simulink model "Mode_plus_Longitudinal"  (R2015a)
settings: Solver=ode45  StartTime=0.0  StopTime=10.0  RelTol=1e-3
undefined symbols (not defined in the file): dt, sample
libraries: simulink x10
settings Model: CovSFcnEnable=off  Creator=teme  LastModifiedBy=teme
settings DataIOCC: SaveFormat=Structure
settings DebuggingCC: UnderspecifiedInitializationDetection=Classic  MergeDetectMultiDrivingBlocksExec=none  SolverPrmCheckMsg=warning  StateNameClashWarn=warning

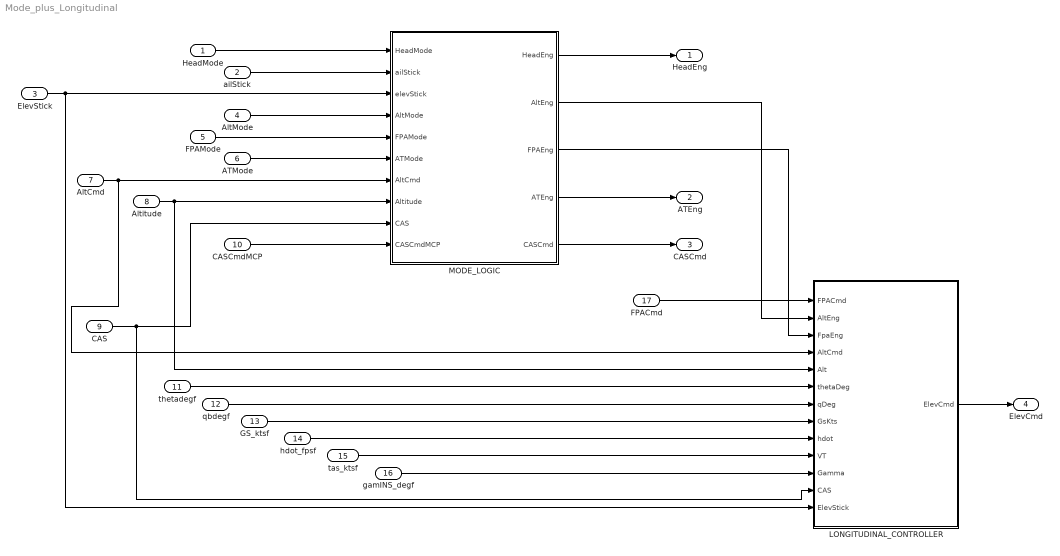
== system Mode_plus_Longitudinal ==
  HeadMode : Inport
  ailStick : Inport  Port=2
  ElevStick : Inport  Port=3
  AltMode : Inport  Port=4
  FPAMode : Inport  Port=5
  ATMode : Inport  Port=6
  AltCmd : Inport  Port=7
  Altitude : Inport  Port=8
  CAS : Inport  Port=9
  CASCmdMCP : Inport  Port=10
  thetadegf : Inport  Port=11  OutDataTypeStr=double
  qbdegf : Inport  Port=12  OutDataTypeStr=double
  GS_ktsf : Inport  Port=13  OutDataTypeStr=double
  "hdot_fpsf " : Inport  Port=14  OutDataTypeStr=double
  tas_ktsf : Inport  Port=15  OutDataTypeStr=double
  gamINS_degf : Inport  Port=16  OutDataTypeStr=double
  FPACmd : Inport  Port=17  OutDataTypeStr=double
  LONGITUDINAL_CONTROLLER : Subsystem  TreatAsAtomicUnit=on
  MODE_LOGIC : Subsystem  TreatAsAtomicUnit=on
  HeadEng : Outport
  ATEng : Outport  Port=2
  CASCmd : Outport  Port=3
  ElevCmd : Outport  RequirementInfo={} %GIDa_1472b341_5948_49bd_8afc_f716c029507f  Port=4
  wires:
  HeadMode/1 -> MODE_LOGIC/1(HeadMode)
  ailStick/1 -> MODE_LOGIC/2(ailStick)
  AltMode/1 -> MODE_LOGIC/4(AltMode)
  FPAMode/1 -> MODE_LOGIC/5(FPAMode)
  ATMode/1 -> MODE_LOGIC/6(ATMode)
  CASCmdMCP/1 -> MODE_LOGIC/10(CASCmdMCP)
  MODE_LOGIC/1(HeadEng) -> HeadEng/1
  MODE_LOGIC/2(AltEng) -> LONGITUDINAL_CONTROLLER/2(AltEng)
  MODE_LOGIC/3(FPAEng) -> LONGITUDINAL_CONTROLLER/3(FpaEng)
  MODE_LOGIC/4(ATEng) -> ATEng/1
  MODE_LOGIC/5(CASCmd) -> CASCmd/1
  LONGITUDINAL_CONTROLLER/1(ElevCmd) -> ElevCmd/1
  CAS/1 -> MODE_LOGIC/9(CAS), LONGITUDINAL_CONTROLLER/12(CAS)
  FPACmd/1 -> LONGITUDINAL_CONTROLLER/1(FPACmd)
  AltCmd/1 -> LONGITUDINAL_CONTROLLER/4(AltCmd), MODE_LOGIC/7(AltCmd)
  Altitude/1 -> MODE_LOGIC/8(Altitude), LONGITUDINAL_CONTROLLER/5(Alt)
  thetadegf/1 -> LONGITUDINAL_CONTROLLER/6(thetaDeg)
  qbdegf/1 -> LONGITUDINAL_CONTROLLER/7(qDeg)
  GS_ktsf/1 -> LONGITUDINAL_CONTROLLER/8(GsKts)
  "hdot_fpsf "/1 -> LONGITUDINAL_CONTROLLER/9(hdot)
  tas_ktsf/1 -> LONGITUDINAL_CONTROLLER/10(VT)
  gamINS_degf/1 -> LONGITUDINAL_CONTROLLER/11(Gamma)
  ElevStick/1 -> LONGITUDINAL_CONTROLLER/13(ElevStick), MODE_LOGIC/3(elevStick)

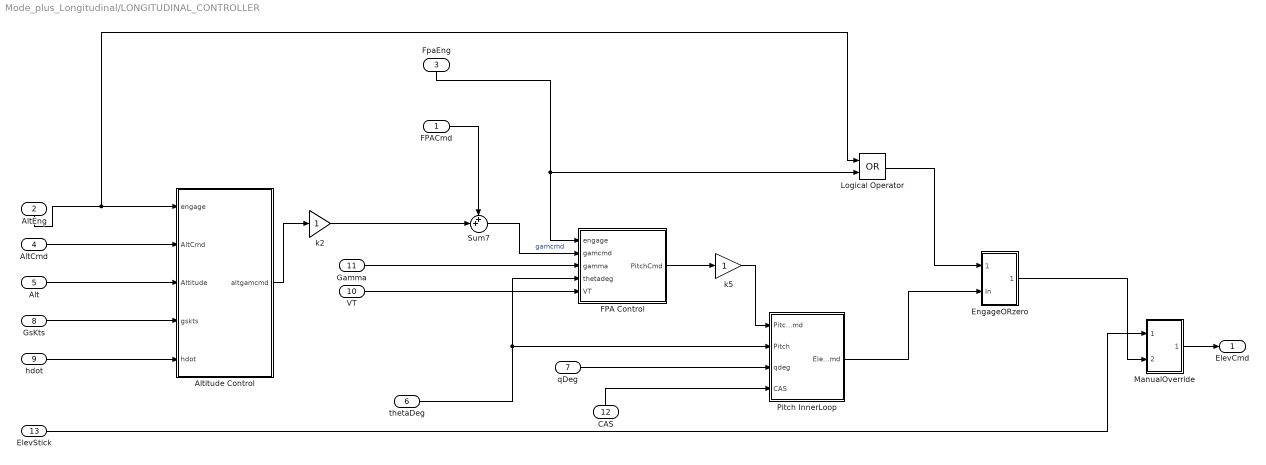
== system Mode_plus_Longitudinal/LONGITUDINAL_CONTROLLER ==
  FPACmd : Inport
  AltEng : Inport  Port=2
  FpaEng : Inport  Port=3
  AltCmd : Inport  Port=4
  Alt : Inport  Port=5
  thetaDeg : Inport  Port=6
  qDeg : Inport  Port=7
  GsKts : Inport  Port=8
  hdot : Inport  Port=9
  VT : Inport  Port=10
  Gamma : Inport  Port=11
  CAS : Inport  Port=12
  ElevStick : Inport  Port=13
  Altitude Control : Subsystem  RequirementInfo={'other' '..\..\tcm_requirements.docx' '@Simulink_requirement_item_14' 'true' 'Altitude Control' '' } %GIDa_355d9ec8_0b7f_4143_baa6_003c4a27f8c0  TreatAsAtomicUnit=on
  EngageORzero : Subsystem  TreatAsAtomicUnit=on
  FPA Control : Subsystem  RequirementInfo={'other' '..\..\tcm_requirements.docx' '@Simulink_requirement_item_15' 'true' 'FPA Control' '' } %GIDa_afe01289_fe8a_4a07_8f72_45e0944c7946  TreatAsAtomicUnit=on
  Logical Operator : Logic  Operator=OR  AllPortsSameDT=off  OutDataTypeStr=boolean
  ManualOverride : Subsystem  TreatAsAtomicUnit=on
  Pitch InnerLoop : Subsystem  RequirementInfo={'other' '..\..\tcm_requirements.docx' '@Simulink_requirement_item_17' 'true' 'Pitch InnerLoop' '' } %GIDa_d1872e6f_e306_4912_a3b7_97524d87ca2c  TreatAsAtomicUnit=on
  Sum7 : Sum  RequirementInfo={} %GIDa_0c140ded_69fd_4573_8acf_9eb9bb189775  Inputs=++|
  k2 : Gain  RequirementInfo={} %GIDa_583ddfee_05b2_4a69_b1d4_b6583806e97d
  k5 : Gain  RequirementInfo={} %GIDa_c5e5a863_50d1_4c0f_a080_0e1eca729c49
  ElevCmd : Outport
  wires:
  k2/1 -> Sum7/2
  Alt/1 -> Altitude Control/3(Altitude)
  thetaDeg/1 -> Pitch InnerLoop/2(Pitch), FPA Control/4(thetadeg)
  Gamma/1 -> FPA Control/3(gamma)
  AltCmd/1 -> Altitude Control/2(AltCmd)
  ManualOverride/1(Out) -> ElevCmd/1
  Altitude Control/1(altgamcmd) -> k2/1
  FPA Control/1(PitchCmd) -> k5/1
  hdot/1 -> Altitude Control/5(hdot)
  Sum7/1 -> FPA Control/2(gamcmd)  "gamcmd"
  qDeg/1 -> Pitch InnerLoop/3(qdeg)
  GsKts/1 -> Altitude Control/4(gskts)
  VT/1 -> FPA Control/5(VT)
  FPACmd/1 -> Sum7/1
  k5/1 -> Pitch InnerLoop/1(PitchCmd)
  FpaEng/1 -> FPA Control/1(engage), Logical Operator/2
  CAS/1 -> Pitch InnerLoop/4(CAS)
  AltEng/1 -> Logical Operator/1, Altitude Control/1(engage)
  ElevStick/1 -> ManualOverride/1(Man)
  Pitch InnerLoop/1(ElevCmd) -> EngageORzero/2(In)
  EngageORzero/1(Out) -> ManualOverride/2(Auto)
  Logical Operator/1 -> EngageORzero/1(Engage)

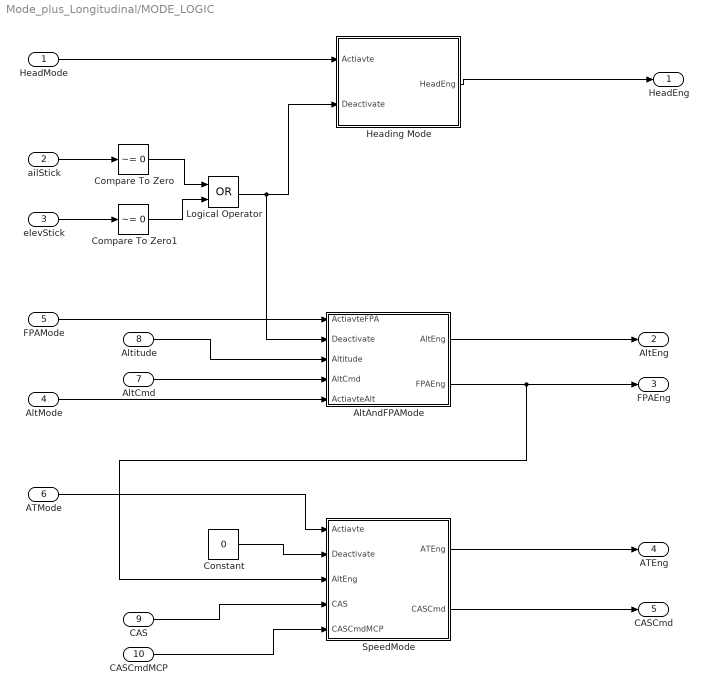
== system Mode_plus_Longitudinal/MODE_LOGIC ==
  HeadMode : Inport
  ailStick : Inport  Port=2
  elevStick : Inport  Port=3
  AltMode : Inport  Port=4
  FPAMode : Inport  Port=5
  ATMode : Inport  Port=6
  AltCmd : Inport  Port=7
  Altitude : Inport  Port=8
  CAS : Inport  Port=9
  CASCmdMCP : Inport  Port=10
  AltAndFPAMode : Subsystem  TreatAsAtomicUnit=on
  Compare To Zero : simulink/Logic and Bit Operations/Compare To Zero  relop=~=  OutDataTypeStr=boolean
  Compare To Zero1 : simulink/Logic and Bit Operations/Compare To Zero  relop=~=  OutDataTypeStr=boolean
  Constant : Constant  Value=0
  Heading Mode : Subsystem  TreatAsAtomicUnit=on
  Logical Operator : Logic  Operator=OR  AllPortsSameDT=off  OutDataTypeStr=boolean
  SpeedMode : Subsystem  TreatAsAtomicUnit=on
  HeadEng : Outport
  AltEng : Outport  Port=2
  FPAEng : Outport  Port=3
  ATEng : Outport  Port=4
  CASCmd : Outport  Port=5
  wires:
  SpeedMode/1(ATEng) -> ATEng/1
  ailStick/1 -> Compare To Zero/1
  Constant/1 -> SpeedMode/2(Deactivate)
  AltAndFPAMode/2(FPAEng) -> FPAEng/1, SpeedMode/3(AltEng)
  AltAndFPAMode/1(AltEng) -> AltEng/1
  Heading Mode/1(HeadEng) -> HeadEng/1
  HeadMode/1 -> Heading Mode/1(Actiavte)
  Compare To Zero1/1 -> Logical Operator/2
  Compare To Zero/1 -> Logical Operator/1
  elevStick/1 -> Compare To Zero1/1
  ATMode/1 -> SpeedMode/1(Actiavte)
  FPAMode/1 -> AltAndFPAMode/1(ActiavteFPA)
  Altitude/1 -> AltAndFPAMode/3(Altitude)
  AltMode/1 -> AltAndFPAMode/5(ActiavteAlt)
  Logical Operator/1 -> AltAndFPAMode/2(Deactivate), Heading Mode/2(Deactivate)
  CASCmdMCP/1 -> SpeedMode/5(CASCmdMCP)
  AltCmd/1 -> AltAndFPAMode/4(AltCmd)
  SpeedMode/2(CASCmd) -> CASCmd/1
  CAS/1 -> SpeedMode/4(CAS)

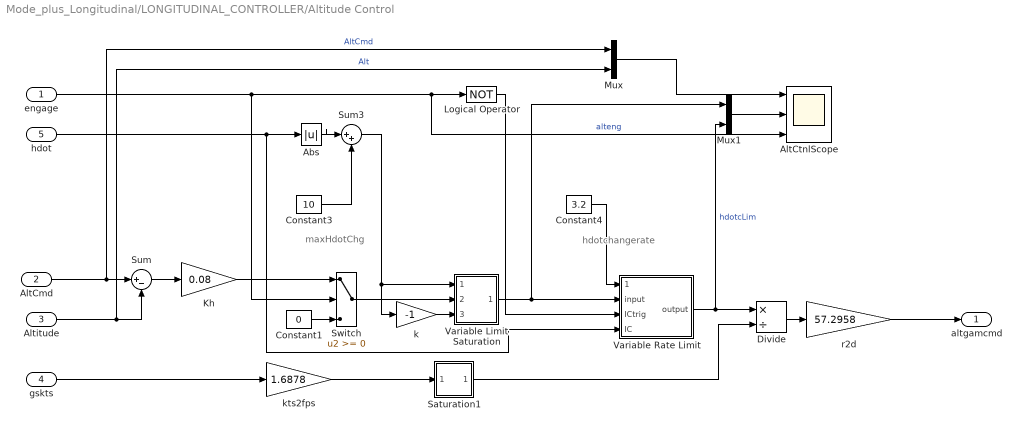
== system Mode_plus_Longitudinal/LONGITUDINAL_CONTROLLER/Altitude Control ==
  note: hdotchangerate
  note: maxHdotChg
  engage : Inport  RequirementInfo={} %GIDa_52c363b5_d7dd_4428_9d3d_bb77c4e76d98
  AltCmd : Inport  RequirementInfo={} %GIDa_0a82d765_f654_4276_830a_f6372a89bbe0  Port=2
  Altitude : Inport  RequirementInfo={} %GIDa_e8d70308_bc0e_4fcb_b765_d7e59f7ec592  Port=3
  gskts : Inport  RequirementInfo={} %GIDa_2af44391_9073_42ae_9a32_99820c2e56f5  Port=4
  hdot : Inport  RequirementInfo={} %GIDa_d9b9fdf0_6dc0_451b_abea_72e0c7ba7654  Port=5
  Abs : Abs  RequirementInfo={} %GIDa_dbe4ef0d_0270_47f9_8208_b0358621302e  SaturateOnIntegerOverflow=on
  AltCtnlScope : Scope  NumInputPorts=3
      settings: RequirementInfo={} %GIDa_cdbaa36f_c6c9_4411_8b52_1b5689d7b849  TimeRange=30  YMin=10000~-5~0  YMax=10200~15~1  SaveName=ScopeData3
  Constant1 : Constant  RequirementInfo={} %GIDa_a96aea24_dc3f_4446_af9b_51dc29300d52  Value=0
  Constant3 : Constant  RequirementInfo={} %GIDa_b1d1ceb1_281f_4f1b_8837_6dd68452e06f  Value=10
  Constant4 : Constant  RequirementInfo={} %GIDa_a7351357_5fac_4e27_bfae_0a136a455002  Value=3.2
  Divide : Product  RequirementInfo={} %GIDa_b8ce34ec_9450_4665_b60e_f19377b61b94  Inputs=*/
  Kh : Gain  RequirementInfo={} %GIDa_2cbc3e69_edde_4cac_a935_06834fe77e88  Gain=0.08
  Logical Operator : Logic  RequirementInfo={} %GIDa_af0e9a41_cde9_4810_9311_1f14359ef5fb  Operator=NOT
  Mux : Mux  RequirementInfo={} %GIDa_47470e8e_2f36_4b9c_b2c4_1f6b7143c7a9  Inputs=2
  Mux1 : Mux  RequirementInfo={} %GIDa_61bb53ed_7736_48c8_9e72_c55612e66728  Inputs=2
  Saturation1 : Subsystem  RequirementInfo={} %GIDa_e76216f3_4aa2_40a0_8972_6dea82147eb2  TreatAsAtomicUnit=on
  Sum : Sum  RequirementInfo={} %GIDa_fdfab13b_0798_40e8_9730_db934c25849e  Inputs=|+-
  Sum3 : Sum  RequirementInfo={} %GIDa_64961105_2569_4900_8a9c_cb8f762adaeb  Inputs=|++  SaturateOnIntegerOverflow=on  InputSameDT=on  OutDataTypeStr=Inherit: Same as first input
  Switch : Switch  RequirementInfo={} %GIDa_2f10cc13_12cd_4e9c_841c_6addbf2a5c41
  Variable Rate Limit : Subsystem  RequirementInfo={} %GIDa_28bb6084_340d_4503_85e9_38193e023d28  TreatAsAtomicUnit=on
  Variable Limit Saturation : Subsystem  RequirementInfo={} %GIDa_69ead1b7_c762_43d5_aef2_f2ccefa8a597  TreatAsAtomicUnit=on
  k : Gain  RequirementInfo={} %GIDa_093f7639_44de_47ca_a1a9_8335a2ae5ad0  Gain=-1
  kts2fps : Gain  RequirementInfo={} %GIDa_c8935b0a_448f_434e_a3c9_42f3e55e9d5b  Gain=1.6878
  r2d : Gain  RequirementInfo={} %GIDa_7be9f1d5_d29b_4985_9ae9_ad523edcc485  Gain=57.2958
  altgamcmd : Outport  RequirementInfo={} %GIDa_a9afaf6f_4f56_4b87_9d4f_e24f69e92c68
  wires:
  Sum/1 -> Kh/1
  AltCmd/1 -> Sum/1, Mux/1  "AltCmd"
  Altitude/1 -> Sum/2, Mux/2  "Alt"
  hdot/1 -> Variable Rate Limit/4(IC), Abs/1
  Abs/1 -> Sum3/1
  Constant3/1 -> Sum3/2
  k/1 -> Variable Limit Saturation/3(Lo_lim)
  Sum3/1 -> k/1, Variable Limit Saturation/1(up_lim)
  engage/1 -> Switch/2, Logical Operator/1, AltCtnlScope/3  "alteng"
  gskts/1 -> kts2fps/1
  Divide/1 -> r2d/1
  r2d/1 -> altgamcmd/1
  Logical Operator/1 -> Variable Rate Limit/3(ICtrig)
  Variable Limit Saturation/1(Out1) -> Variable Rate Limit/2(input), Mux1/1
  Constant4/1 -> Variable Rate Limit/1(ratelim)
  Variable Rate Limit/1(output) -> Divide/1, Mux1/2  "hdotcLim"
  kts2fps/1 -> Saturation1/1(SigIn)
  Saturation1/1(Out1) -> Divide/2
  Switch/1 -> Variable Limit Saturation/2(SigIn)
  Kh/1 -> Switch/1
  Constant1/1 -> Switch/3
  Mux/1 -> AltCtnlScope/1
  Mux1/1 -> AltCtnlScope/2

== system Mode_plus_Longitudinal/LONGITUDINAL_CONTROLLER/EngageORzero ==
  Engage : Inport
  In : Inport  Port=2
  Logical Operator5 : Logic  RequirementInfo={} %GIDa_ccfc23e2_0411_4b04_aca7_2de4f158b6cd  AllPortsSameDT=off  OutDataTypeStr=boolean
  Switch1 : Switch  RequirementInfo={} %GIDa_254e92ee_ae0a_4bfe_bfdb_e4c06df78b5d  Threshold=0.5
  zero10 : Constant  RequirementInfo={} %GIDa_d207173f_5f9f_4849_a51b_8675c5c4c9c2
  zero9 : Constant  RequirementInfo={} %GIDa_ffbd3266_7e8f_4b22_959a_f4ffeace0558  Value=0
  Out : Outport
  wires:
  Engage/1 -> Logical Operator5/1
  zero10/1 -> Logical Operator5/2
  zero9/1 -> Switch1/3
  In/1 -> Switch1/1
  Logical Operator5/1 -> Switch1/2
  Switch1/1 -> Out/1

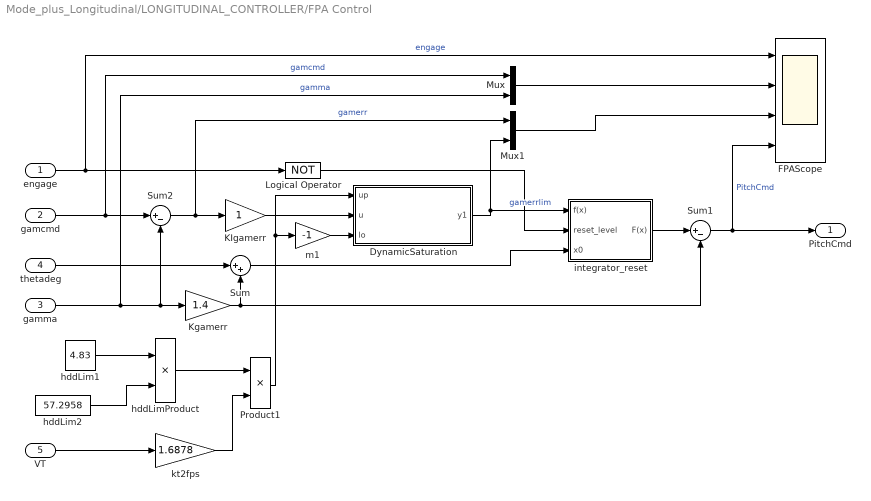
== system Mode_plus_Longitudinal/LONGITUDINAL_CONTROLLER/FPA Control ==
  engage : Inport  RequirementInfo={} %GIDa_a5ca5c72_1624_4f57_8848_6838dbeb69e5  OutDataTypeStr=boolean
  gamcmd : Inport  RequirementInfo={} %GIDa_f539d9e5_1422_4ddf_9938_0897544f30cd  Port=2  OutDataTypeStr=double
  gamma : Inport  RequirementInfo={} %GIDa_e241222a_57fb_4f96_ba9f_1fd449c16db7  Port=3  OutDataTypeStr=double
  thetadeg : Inport  RequirementInfo={} %GIDa_3c46ec82_f68a_45df_8609_de83facd241a  Port=4  OutDataTypeStr=double
  VT : Inport  RequirementInfo={} %GIDa_d515a720_002f_4829_a2a6_18045b0ac777  Port=5  OutDataTypeStr=double
  DynamicSaturation : Subsystem  TreatAsAtomicUnit=on
  FPAScope : Scope  NumInputPorts=4
      settings: RequirementInfo={} %GIDa_7cc530c8_9ccc_4bfe_b80a_f4375f56bd14  YMin=-1~-5~-2~-5  YMax=2~5~2~10
  KIgamerr : Gain  RequirementInfo={} %GIDa_82260f55_a1de_42fb_b735_9e4599f81841
  Kgamerr : Gain  RequirementInfo={} %GIDa_16083332_5456_45f2_a369_a033765805fc  Gain=1.4
  Logical Operator : Logic  RequirementInfo={} %GIDa_f4beb439_5138_4af2_9bd0_3d7cb852e6ec  Operator=NOT  AllPortsSameDT=off  OutDataTypeStr=boolean
  Mux : Mux  RequirementInfo={} %GIDa_f4a4be95_68e7_4fcc_80ef_d6f12325c5c6  Inputs=2
  Mux1 : Mux  RequirementInfo={} %GIDa_856a70e5_571d_4800_b63e_8744bb9a992b  Inputs=2
  Product1 : Product  RequirementInfo={} %GIDa_8e2f5a82_1404_4ef2_8700_b1676a09c733  RndMeth=Zero
  Sum : Sum  RequirementInfo={} %GIDa_2c46e54a_16c3_48c1_a530_4e77b3b6f7cf  Inputs=|++
  Sum1 : Sum  RequirementInfo={} %GIDa_5447bb63_ee33_484d_a3fb_66639f30e65e  Inputs=|+-
  Sum2 : Sum  RequirementInfo={} %GIDa_e6a645c9_6b06_4015_88ce_f90087de6b14  Inputs=|+-
  hddLim1 : Constant  Value=4.83  SampleTime=sample
  hddLim2 : Constant  Value=57.2958  SampleTime=sample
  hddLimProduct : Product  RndMeth=Zero
  integrator_reset : Subsystem  TreatAsAtomicUnit=on
  kt2fps : Gain  RequirementInfo={} %GIDa_e958a29f_6566_4fb6_a607_06b409395c8a  Gain=1.6878
  m1 : Gain  RequirementInfo={} %GIDa_f600f599_b9eb_4aa5_a121_c23ac8246818  Gain=-1
  PitchCmd : Outport  RequirementInfo={} %GIDa_7642116b_0bfd_4af5_a213_a8cf8bf5662a  OutDataTypeStr=double
  wires:
  Sum1/1 -> PitchCmd/1, FPAScope/4  "PitchCmd"
  Kgamerr/1 -> Sum1/2, Sum/2
  integrator_reset/1(F(x)) -> Sum1/1
  gamma/1 -> Kgamerr/1, Sum2/2, Mux/2  "gamma"
  thetadeg/1 -> Sum/1
  Sum/1 -> integrator_reset/3(x0)
  engage/1 -> Logical Operator/1, FPAScope/1  "engage"
  Logical Operator/1 -> integrator_reset/2(reset_level)
  kt2fps/1 -> Product1/2
  hddLimProduct/1 -> Product1/1
  Product1/1 -> m1/1, DynamicSaturation/1(up)
  VT/1 -> kt2fps/1
  DynamicSaturation/1(y1) -> integrator_reset/1(f(x)), Mux1/2  "gamerrlim"
  KIgamerr/1 -> DynamicSaturation/2(u)
  m1/1 -> DynamicSaturation/3(lo)
  Sum2/1 -> KIgamerr/1, Mux1/1  "gamerr"
  gamcmd/1 -> Sum2/1, Mux/1  "gamcmd"
  Mux/1 -> FPAScope/2
  Mux1/1 -> FPAScope/3
  hddLim1/1 -> hddLimProduct/1
  hddLim2/1 -> hddLimProduct/2

== system Mode_plus_Longitudinal/LONGITUDINAL_CONTROLLER/ManualOverride ==
  Man : Inport
  Auto : Inport  Port=2
  Switch1 : Switch  RequirementInfo={} %GIDa_69cd44cc_695c_4e4c_b729_5e76b03a5c9b  Criteria=u2 ~= 0  Threshold=0.5
  Out : Outport
  wires:
  Man/1 -> Switch1/3, Switch1/2
  Auto/1 -> Switch1/1
  Switch1/1 -> Out/1

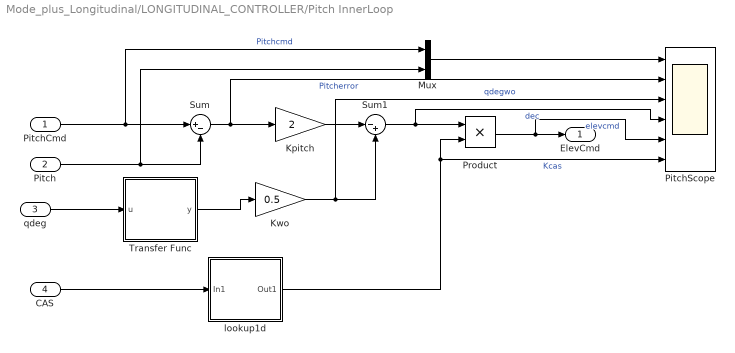
== system Mode_plus_Longitudinal/LONGITUDINAL_CONTROLLER/Pitch InnerLoop ==
  PitchCmd : Inport  RequirementInfo={} %GIDa_2fa8ae42_3276_495e_b4da_5cc7558fe53e  OutDataTypeStr=double
  Pitch : Inport  RequirementInfo={} %GIDa_e0b05770_7d89_48ca_ae42_7e8bc3cf70e1  Port=2  OutDataTypeStr=double
  qdeg : Inport  RequirementInfo={} %GIDa_32a3f04f_fa35_48b7_ae05_62ba74ce8106  Port=3  OutDataTypeStr=double
  CAS : Inport  RequirementInfo={} %GIDa_376f2873_f9f7_4b29_ab34_f3040502ee08  Port=4  OutDataTypeStr=double
  Kpitch : Gain  RequirementInfo={} %GIDa_7fbbd552_ea5b_4045_aa48_b875de2b9e68  Gain=2
  Kwo : Gain  RequirementInfo={} %GIDa_e54031bb_ac6b_45ac_907a_c4f2d5dd216d  Gain=0.5
  Mux : Mux  RequirementInfo={} %GIDa_2fd7bb9e_bac2_4662_8409_53cd9298505a  Inputs=2
  PitchScope : Scope  NumInputPorts=6
      settings: RequirementInfo={} %GIDa_582b22f1_949b_4cc3_a4ef_9b9996bc8938  YMin=-2~-2~-2~-20~-20~0  YMax=10~2~2~20~20~1.2  SaveName=ScopeData2
  Product : Product  RequirementInfo={} %GIDa_c4cbe03c_2c4b_4cd5_b1a2_997256c1b301  RndMeth=Zero
  Sum : Sum  RequirementInfo={} %GIDa_7f5d0d6d_f9e4_4238_a87c_9ed250c3eb97  Inputs=|+-
  Sum1 : Sum  RequirementInfo={} %GIDa_de0046de_cb27_4b4c_8300_061022f2300c  Inputs=|-+
  Transfer Func : Subsystem  TreatAsAtomicUnit=on
  lookup1d : Subsystem  TreatAsAtomicUnit=on
  ElevCmd : Outport  RequirementInfo={} %GIDa_3f515e46_808e_46ad_97d1_bb9b634324b0
  wires:
  Sum/1 -> Kpitch/1, PitchScope/2  "Pitcherror"
  Pitch/1 -> Sum/2, Mux/2
  Kpitch/1 -> Sum1/1
  qdeg/1 -> Transfer Func/1(u)
  Transfer Func/1(y) -> Kwo/1
  CAS/1 -> lookup1d/1(In1)
  Sum1/1 -> Product/1, PitchScope/4  "dec"
  lookup1d/1(Out1) -> Product/2, PitchScope/6  "Kcas"
  Product/1 -> ElevCmd/1, PitchScope/5  "elevcmd"
  Kwo/1 -> Sum1/2, PitchScope/3  "qdegwo"
  PitchCmd/1 -> Sum/1, Mux/1  "Pitchcmd"
  Mux/1 -> PitchScope/1

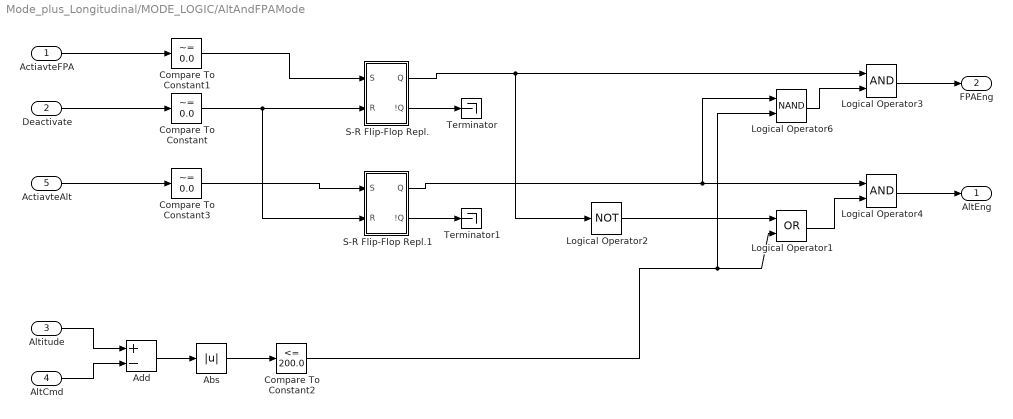
== system Mode_plus_Longitudinal/MODE_LOGIC/AltAndFPAMode ==
  ActiavteFPA : Inport
  Deactivate : Inport  Port=2
  Altitude : Inport  Port=3
  AltCmd : Inport  Port=4
  ActiavteAlt : Inport  Port=5
  Abs : Abs
  Add : Sum  Inputs=+-
  Compare To Constant : simulink/Logic and Bit Operations/Compare To Constant  relop=~=  const=0.0  OutDataTypeStr=boolean
  Compare To Constant1 : simulink/Logic and Bit Operations/Compare To Constant  relop=~=  const=0.0  OutDataTypeStr=boolean
  Compare To Constant2 : simulink/Logic and Bit Operations/Compare To Constant  relop=<=  const=200.0  OutDataTypeStr=boolean
  Compare To Constant3 : simulink/Logic and Bit Operations/Compare To Constant  relop=~=  const=0.0  OutDataTypeStr=boolean
  Logical Operator1 : Logic  Operator=OR  AllPortsSameDT=off  OutDataTypeStr=boolean
  Logical Operator2 : Logic  Operator=NOT  AllPortsSameDT=off  OutDataTypeStr=boolean
  Logical Operator3 : Logic  AllPortsSameDT=off  OutDataTypeStr=boolean
  Logical Operator4 : Logic  AllPortsSameDT=off  OutDataTypeStr=boolean
  Logical Operator6 : Logic  Operator=NAND  AllPortsSameDT=off  OutDataTypeStr=boolean
  S-R Flip-Flop Repl. : Subsystem
  S-R Flip-Flop Repl.1 : Subsystem
  Terminator : Terminator
  Terminator1 : Terminator
  AltEng : Outport
  FPAEng : Outport  Port=2
  wires:
  S-R Flip-Flop Repl./2(!Q) -> Terminator/1
  ActiavteFPA/1 -> Compare To Constant1/1
  S-R Flip-Flop Repl./1(Q) -> Logical Operator3/1, Logical Operator2/1
  Deactivate/1 -> Compare To Constant/1
  Compare To Constant1/1 -> S-R Flip-Flop Repl./1(S)
  S-R Flip-Flop Repl.1/2(!Q) -> Terminator1/1
  S-R Flip-Flop Repl.1/1(Q) -> Logical Operator6/1, Logical Operator4/1
  Compare To Constant3/1 -> S-R Flip-Flop Repl.1/1(S)
  Compare To Constant/1 -> S-R Flip-Flop Repl.1/2(R), S-R Flip-Flop Repl./2(R)
  ActiavteAlt/1 -> Compare To Constant3/1
  Altitude/1 -> Add/1
  AltCmd/1 -> Add/2
  Add/1 -> Abs/1
  Abs/1 -> Compare To Constant2/1
  Logical Operator3/1 -> FPAEng/1
  Logical Operator2/1 -> Logical Operator1/1
  Logical Operator4/1 -> AltEng/1
  Compare To Constant2/1 -> Logical Operator6/2, Logical Operator1/2
  Logical Operator1/1 -> Logical Operator4/2
  Logical Operator6/1 -> Logical Operator3/2

== system Mode_plus_Longitudinal/MODE_LOGIC/Heading Mode ==
  Actiavte : Inport
  Deactivate : Inport  Port=2
  Compare To Constant : simulink/Logic and Bit Operations/Compare To Constant  relop=~=  const=0.0  OutDataTypeStr=boolean
  Compare To Constant1 : simulink/Logic and Bit Operations/Compare To Constant  relop=~=  const=0.0  OutDataTypeStr=boolean
  S-R Flip-Flop Repl. : Subsystem
  Terminator : Terminator
  HeadEng : Outport
  wires:
  S-R Flip-Flop Repl./2(!Q) -> Terminator/1
  Actiavte/1 -> Compare To Constant1/1
  S-R Flip-Flop Repl./1(Q) -> HeadEng/1
  Deactivate/1 -> Compare To Constant/1
  Compare To Constant1/1 -> S-R Flip-Flop Repl./1(S)
  Compare To Constant/1 -> S-R Flip-Flop Repl./2(R)

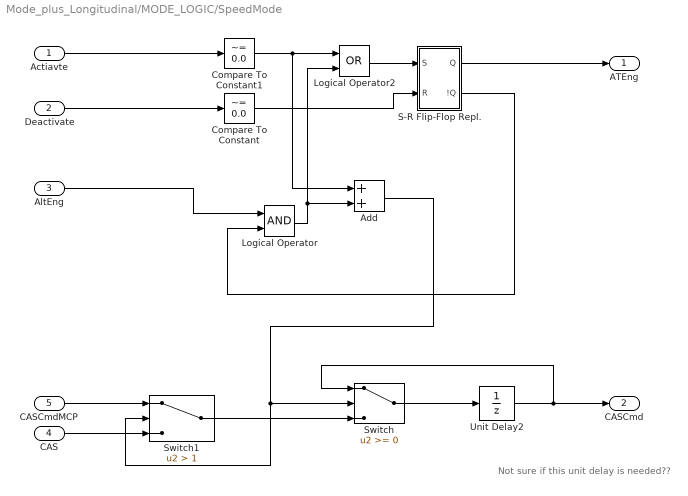
== system Mode_plus_Longitudinal/MODE_LOGIC/SpeedMode ==
  note: Not sure if this unit delay is needed??
  Actiavte : Inport
  Deactivate : Inport  Port=2
  AltEng : Inport  Port=3
  CAS : Inport  Port=4
  CASCmdMCP : Inport  Port=5
  Add : Sum
  Compare To Constant : simulink/Logic and Bit Operations/Compare To Constant  relop=~=  const=0.0  OutDataTypeStr=boolean
  Compare To Constant1 : simulink/Logic and Bit Operations/Compare To Constant  relop=~=  const=0.0  OutDataTypeStr=boolean
  Logical Operator : Logic  AllPortsSameDT=off  OutDataTypeStr=boolean
  Logical Operator2 : Logic  Operator=OR  AllPortsSameDT=off  OutDataTypeStr=boolean
  S-R Flip-Flop Repl. : Subsystem
  Switch : Switch
  Switch1 : Switch  Criteria=u2 > Threshold  Threshold=1
  Unit Delay2 : UnitDelay  SampleTime=-1
  ATEng : Outport
  CASCmd : Outport  Port=2
  wires:
  Actiavte/1 -> Compare To Constant1/1
  S-R Flip-Flop Repl./1(Q) -> ATEng/1
  Deactivate/1 -> Compare To Constant/1
  Compare To Constant/1 -> S-R Flip-Flop Repl./2(R)
  AltEng/1 -> Logical Operator/1
  Logical Operator2/1 -> S-R Flip-Flop Repl./1(S)
  Logical Operator/1 -> Add/2, Logical Operator2/2
  CAS/1 -> Switch1/3
  CASCmdMCP/1 -> Switch1/1
  Compare To Constant1/1 -> Add/1, Logical Operator2/1
  Add/1 -> Switch1/2, Switch/2
  Switch1/1 -> Switch/3
  Switch/1 -> Unit Delay2/1
  Unit Delay2/1 -> Switch/1, CASCmd/1
  S-R Flip-Flop Repl./2(!Q) -> Logical Operator/2

== system Mode_plus_Longitudinal/LONGITUDINAL_CONTROLLER/Altitude Control/Saturation1 ==
  SigIn : Inport  RequirementInfo={} %GIDa_ad3eafa4_8ac6_497c_88bd_c56259265039
  Constant1 : Constant  RequirementInfo={} %GIDa_95510516_d7e2_4fd7_b056_b2d217454ab2  Value=0.0001
  Constant2 : Constant  RequirementInfo={} %GIDa_3cd71bdc_2b02_4615_b303_cb043727f9a9  Value=1000
  Enforce low lim : MinMax  RequirementInfo={} %GIDa_7efad45a_619a_4d3d_82f0_d07bdc6d10c7  Function=max  Inputs=2
  Enforce up lim : MinMax  RequirementInfo={} %GIDa_b14da782_d71e_4362_9ffc_9cadb2230f1f  Inputs=2
  Out1 : Outport  RequirementInfo={} %GIDa_ecc04fbc_b892_46b6_9eeb_812fbd261572
  wires:
  Constant1/1 -> Enforce low lim/1
  SigIn/1 -> Enforce low lim/2
  Enforce low lim/1 -> Enforce up lim/1
  Constant2/1 -> Enforce up lim/2
  Enforce up lim/1 -> Out1/1

== system Mode_plus_Longitudinal/LONGITUDINAL_CONTROLLER/Altitude Control/Variable Rate Limit ==
  ratelim : Inport  RequirementInfo={} %GIDa_9884ed4f_54b8_4838_a590_2f1197ef9d03
  input : Inport  RequirementInfo={} %GIDa_907ac359_721f_42d4_b7f1_2a5095e0076d  Port=2  OutDataTypeStr=double
  ICtrig : Inport  RequirementInfo={} %GIDa_4962c24b_3968_4eab_8798_02644b9819ea  Port=3
  IC : Inport  RequirementInfo={} %GIDa_09cf7c58_4c94_43aa_b076_301358e60b57  Port=4
  Gain : Gain  RequirementInfo={} %GIDa_394274d4_9872_40e2_ab5c_6354650f6cb1  Gain=20  SaturateOnIntegerOverflow=on  OutDataTypeStr=Inherit: Same as input  ParamDataTypeStr=Inherit: Same as input
  Gain1 : Gain  RequirementInfo={} %GIDa_2fb6f3ea_d5dd_4654_ad59_cfb73cb6d460  Gain=-1  SaturateOnIntegerOverflow=on  OutDataTypeStr=Inherit: Same as input  ParamDataTypeStr=Inherit: Same as input
  Sum2 : Sum  RequirementInfo={} %GIDa_750a5874_9618_4084_a68e_7eb74d6028a6  Inputs=|+-  SaturateOnIntegerOverflow=on
  Variable Limit Saturation : Subsystem  RequirementInfo={} %GIDa_3eb72791_134a_4333_b2be_8b66f1f8df20  TreatAsAtomicUnit=on
  integrator_reset : Subsystem
  output : Outport  RequirementInfo={} %GIDa_ab95990d_3762_49ec_8191_f2a1d00afca9
  wires:
  Sum2/1 -> Gain/1
  Gain/1 -> Variable Limit Saturation/2(SigIn)
  ratelim/1 -> Gain1/1, Variable Limit Saturation/1(up_lim)
  Gain1/1 -> Variable Limit Saturation/3(Lo_lim)
  integrator_reset/1(F(x)) -> Sum2/2, output/1
  input/1 -> Sum2/1
  ICtrig/1 -> integrator_reset/2(reset_level)
  IC/1 -> integrator_reset/3(x0)
  Variable Limit Saturation/1(Out1) -> integrator_reset/1(f(x))

== system Mode_plus_Longitudinal/LONGITUDINAL_CONTROLLER/Altitude Control/Variable Limit Saturation ==
  up_lim : Inport  RequirementInfo={} %GIDa_99cabfbf_efdf_4db1_a654_cf9a8823f13a
  SigIn : Inport  RequirementInfo={} %GIDa_e45d4aa8_7b1e_4db6_bd7a_e9c2c8461fd1  Port=2
  Lo_lim : Inport  RequirementInfo={} %GIDa_609fc770_0241_4e24_8e13_af8b47c08b7d  Port=3
  Enforce low lim : MinMax  RequirementInfo={} %GIDa_f4ceb581_e70d_4aa0_b4b6_141d717964fd  Function=max  Inputs=2
  Enforce up lim : MinMax  RequirementInfo={} %GIDa_ed56a3e2_0853_443a_b92a_28eb249b6a33  Inputs=2
  Out1 : Outport  RequirementInfo={} %GIDa_bd35131e_df1f_41fa_9f2f_140173596c7d
  wires:
  Lo_lim/1 -> Enforce low lim/1
  SigIn/1 -> Enforce low lim/2
  Enforce low lim/1 -> Enforce up lim/1
  up_lim/1 -> Enforce up lim/2
  Enforce up lim/1 -> Out1/1

== system Mode_plus_Longitudinal/LONGITUDINAL_CONTROLLER/FPA Control/DynamicSaturation ==
  up : Inport
  u : Inport  Port=2
  lo : Inport  Port=3
  LowerRelop1 : RelationalOperator  DisableCoverage=on  Operator=>  OutDataTypeStr=boolean
  Switch : Switch  Criteria=u2 ~= 0  OutDataTypeStr=Inherit: Inherit via back propagation  ZeroCross=off
  Switch2 : Switch  Criteria=u2 ~= 0  OutDataTypeStr=Inherit: Inherit via back propagation  ZeroCross=off
  UpperRelop : RelationalOperator  DisableCoverage=on  Operator=<  OutDataTypeStr=boolean
  y1 : Outport
  wires:
  up/1 -> Switch2/1, LowerRelop1/2
  u/1 -> Switch/3, LowerRelop1/1, UpperRelop/1
  lo/1 -> Switch/1, UpperRelop/2
  Switch/1 -> Switch2/3
  Switch2/1 -> y1/1
  LowerRelop1/1 -> Switch2/2
  UpperRelop/1 -> Switch/2

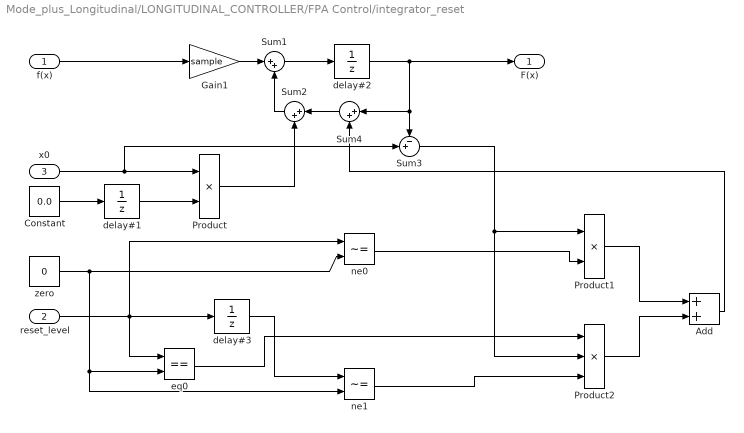
== system Mode_plus_Longitudinal/LONGITUDINAL_CONTROLLER/FPA Control/integrator_reset ==
  f(x) : Inport
  reset_level : Inport  Port=2
  x0 : Inport  Port=3
  Add : Sum
  Constant : Constant  Value=0.0  SampleTime=sample
  Gain1 : Gain  RequirementInfo={} %GIDa_5239248c_eaee_4a86_8425_3843d2c23e6f  Gain=sample
  Product : Product  RndMeth=Zero
  Product1 : Product  RndMeth=Zero
  Product2 : Product  Inputs=3  RndMeth=Zero
  Sum1 : Sum  RequirementInfo={} %GIDa_572bc924_1f7b_4505_b080_8fbc2ab696a1  Inputs=|++
  Sum2 : Sum  RequirementInfo={} %GIDa_d01c2530_10bd_4e38_9a4f_f370db915155  Inputs=|++
  Sum3 : Sum  RequirementInfo={} %GIDa_343fb48c_21b6_4ee0_9c9c_cbeff0735f27  Inputs=-+|
  Sum4 : Sum  RequirementInfo={} %GIDa_f5b18c8b_35f1_44ae_b108_9529fe738422  Inputs=|++
  delay#1 : UnitDelay  InitialCondition=1.0  SampleTime=-1
  delay#2 : UnitDelay  InitialCondition=0.0  SampleTime=-1
  delay#3 : UnitDelay  InitialCondition=0.0  SampleTime=-1
  eq0 : RelationalOperator  Operator===  OutDataTypeStr=boolean
  ne0 : RelationalOperator  Operator=~=  OutDataTypeStr=boolean
  ne1 : RelationalOperator  Operator=~=  OutDataTypeStr=boolean
  zero : Constant  Value=0  SampleTime=sample
  F(x) : Outport  RequirementInfo={} %GIDa_1c97e49d_b0d4_4d64_849e_02e72b937e8d
  wires:
  Sum1/1 -> delay#2/1
  Gain1/1 -> Sum1/1
  delay#2/1 -> F(x)/1, Sum3/1, Sum4/1
  Sum2/1 -> Sum1/2
  Product/1 -> Sum2/2
  delay#1/1 -> Product/2
  Constant/1 -> delay#1/1
  f(x)/1 -> Gain1/1
  x0/1 -> Product/1, Sum3/2
  reset_level/1 -> delay#3/1, ne0/1, eq0/1
  delay#3/1 -> ne1/1
  Sum3/1 -> Product1/1, Product2/2
  ne0/1 -> Product1/2
  eq0/1 -> Product2/1
  Product1/1 -> Add/1
  Product2/1 -> Add/2
  zero/1 -> ne0/2, eq0/2, ne1/2
  ne1/1 -> Product2/3
  Sum4/1 -> Sum2/1
  Add/1 -> Sum4/2

== system Mode_plus_Longitudinal/LONGITUDINAL_CONTROLLER/Pitch InnerLoop/Transfer Func ==
  u : Inport  OutDataTypeStr=double  PortDimensions=1  SampleTime=dt
  a#1 : Gain  Gain=0.0625
  b0#0 : Gain
  b0#1 : Gain  Gain=-1
  delay#1 : UnitDelay  InitialCondition=0.0  SampleTime=-1
  output_sum : Sum
  sample#1 : Gain  Gain=0.02
  sum11 : Sum  Inputs=|+-
  sum21 : Sum  Inputs=|++
  y : Outport
  wires:
  delay#1/1 -> a#1/1, sum21/2
  a#1/1 -> sum11/2, b0#1/1
  b0#0/1 -> output_sum/1
  b0#1/1 -> output_sum/2
  sum11/1 -> sample#1/1
  sample#1/1 -> sum21/1
  sum21/1 -> delay#1/1
  u/1 -> sum11/1, b0#0/1
  output_sum/1 -> y/1

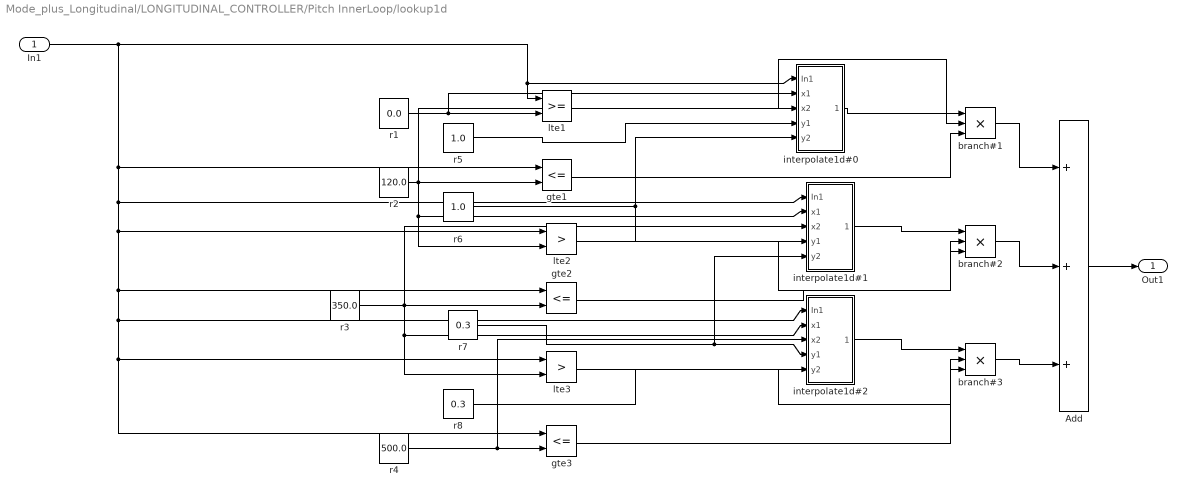
== system Mode_plus_Longitudinal/LONGITUDINAL_CONTROLLER/Pitch InnerLoop/lookup1d ==
  In1 : Inport  OutDataTypeStr=double
  Add : Sum  Inputs=+++
  branch#1 : Product  Inputs=3  RndMeth=Zero
  branch#2 : Product  Inputs=3  RndMeth=Zero
  branch#3 : Product  Inputs=3  RndMeth=Zero
  gte1 : RelationalOperator  Operator=<=  OutDataTypeStr=boolean  SampleTime=sample
  gte2 : RelationalOperator  Operator=<=  OutDataTypeStr=boolean  SampleTime=sample
  gte3 : RelationalOperator  Operator=<=  OutDataTypeStr=boolean  SampleTime=sample
  interpolate1d#0 : Subsystem  TreatAsAtomicUnit=on
  interpolate1d#1 : Subsystem  TreatAsAtomicUnit=on
  interpolate1d#2 : Subsystem  TreatAsAtomicUnit=on
  lte1 : RelationalOperator  OutDataTypeStr=boolean
  lte2 : RelationalOperator  Operator=>  OutDataTypeStr=boolean
  lte3 : RelationalOperator  Operator=>  OutDataTypeStr=boolean
  r1 : Constant  Value=0.0  SampleTime=sample
  r2 : Constant  Value=120.0  SampleTime=sample
  r3 : Constant  Value=350.0  SampleTime=sample
  r4 : Constant  Value=500.0  SampleTime=sample
  r5 : Constant  Value=1.0  SampleTime=sample
  r6 : Constant  Value=1.0  SampleTime=sample
  r7 : Constant  Value=0.3  SampleTime=sample
  r8 : Constant  Value=0.3  SampleTime=sample
  Out1 : Outport
  wires:
  r4/1 -> gte3/2, interpolate1d#2/3(x2)
  r3/1 -> gte2/2, interpolate1d#1/3(x2), lte3/2, interpolate1d#2/2(x1)
  r2/1 -> gte1/2, interpolate1d#0/3(x2), lte2/2, interpolate1d#1/2(x1)
  r1/1 -> lte1/2, interpolate1d#0/2(x1)
  In1/1 -> gte1/1, lte2/1, gte2/1, lte3/1, gte3/1, interpolate1d#2/1(In1), interpolate1d#1/1(In1), lte1/1, interpolate1d#0/1(In1)
  interpolate1d#0/1(Out1) -> branch#1/1
  r8/1 -> interpolate1d#2/5(y2)
  r7/1 -> interpolate1d#2/4(y1), interpolate1d#1/5(y2)
  r6/1 -> interpolate1d#1/4(y1), interpolate1d#0/5(y2)
  r5/1 -> interpolate1d#0/4(y1)
  interpolate1d#2/1(Out1) -> branch#3/1
  interpolate1d#1/1(Out1) -> branch#2/1
  lte1/1 -> branch#1/2
  gte1/1 -> branch#1/3
  lte2/1 -> branch#2/2
  gte2/1 -> branch#2/3
  lte3/1 -> branch#3/2
  gte3/1 -> branch#3/3
  branch#1/1 -> Add/1
  branch#2/1 -> Add/2
  branch#3/1 -> Add/3
  Add/1 -> Out1/1

== system Mode_plus_Longitudinal/MODE_LOGIC/AltAndFPAMode/S-R Flip-Flop Repl. ==
  S : Inport
  R : Inport  Port=2
  Logical Operator : Logic  Operator=NAND  AllPortsSameDT=off  OutDataTypeStr=boolean
  Logical Operator1 : Logic  Operator=NAND  AllPortsSameDT=off  OutDataTypeStr=boolean
  Logical Operator2 : Logic  Operator=NOT  AllPortsSameDT=off  OutDataTypeStr=boolean
  Logical Operator3 : Logic  Operator=NOT  AllPortsSameDT=off  OutDataTypeStr=boolean
  Unit Delay : UnitDelay  SampleTime=-1
  Unit Delay1 : UnitDelay  InitialCondition=1  SampleTime=-1
  Q : Outport
  !Q : Outport  Port=2
  wires:
  Logical Operator/1 -> Unit Delay1/1, !Q/1
  Logical Operator1/1 -> Unit Delay/1, Q/1
  Unit Delay/1 -> Logical Operator/1
  Unit Delay1/1 -> Logical Operator1/2
  Logical Operator2/1 -> Logical Operator1/1
  Logical Operator3/1 -> Logical Operator/2
  R/1 -> Logical Operator3/1
  S/1 -> Logical Operator2/1

== system Mode_plus_Longitudinal/MODE_LOGIC/AltAndFPAMode/S-R Flip-Flop Repl.1 ==
  S : Inport
  R : Inport  Port=2
  Logical Operator : Logic  Operator=NAND  AllPortsSameDT=off  OutDataTypeStr=boolean
  Logical Operator1 : Logic  Operator=NAND  AllPortsSameDT=off  OutDataTypeStr=boolean
  Logical Operator2 : Logic  Operator=NOT  AllPortsSameDT=off  OutDataTypeStr=boolean
  Logical Operator3 : Logic  Operator=NOT  AllPortsSameDT=off  OutDataTypeStr=boolean
  Unit Delay : UnitDelay  SampleTime=-1
  Unit Delay1 : UnitDelay  InitialCondition=1  SampleTime=-1
  Q : Outport
  !Q : Outport  Port=2
  wires:
  Logical Operator/1 -> Unit Delay1/1, !Q/1
  Logical Operator1/1 -> Unit Delay/1, Q/1
  Unit Delay/1 -> Logical Operator/1
  Unit Delay1/1 -> Logical Operator1/2
  Logical Operator2/1 -> Logical Operator1/1
  Logical Operator3/1 -> Logical Operator/2
  R/1 -> Logical Operator3/1
  S/1 -> Logical Operator2/1

== system Mode_plus_Longitudinal/MODE_LOGIC/Heading Mode/S-R Flip-Flop Repl. ==
  S : Inport
  R : Inport  Port=2
  Logical Operator : Logic  Operator=NAND  AllPortsSameDT=off  OutDataTypeStr=boolean
  Logical Operator1 : Logic  Operator=NAND  AllPortsSameDT=off  OutDataTypeStr=boolean
  Logical Operator2 : Logic  Operator=NOT  AllPortsSameDT=off  OutDataTypeStr=boolean
  Logical Operator3 : Logic  Operator=NOT  AllPortsSameDT=off  OutDataTypeStr=boolean
  Unit Delay : UnitDelay  SampleTime=-1
  Unit Delay1 : UnitDelay  InitialCondition=1  SampleTime=-1
  Q : Outport
  !Q : Outport  Port=2
  wires:
  Logical Operator/1 -> Unit Delay1/1, !Q/1
  Logical Operator1/1 -> Unit Delay/1, Q/1
  Unit Delay/1 -> Logical Operator/1
  Unit Delay1/1 -> Logical Operator1/2
  Logical Operator2/1 -> Logical Operator1/1
  Logical Operator3/1 -> Logical Operator/2
  R/1 -> Logical Operator3/1
  S/1 -> Logical Operator2/1

== system Mode_plus_Longitudinal/MODE_LOGIC/SpeedMode/S-R Flip-Flop Repl. ==
  S : Inport
  R : Inport  Port=2
  Logical Operator : Logic  Operator=NAND  AllPortsSameDT=off  OutDataTypeStr=boolean
  Logical Operator1 : Logic  Operator=NAND  AllPortsSameDT=off  OutDataTypeStr=boolean
  Logical Operator2 : Logic  Operator=NOT  AllPortsSameDT=off  OutDataTypeStr=boolean
  Logical Operator3 : Logic  Operator=NOT  AllPortsSameDT=off  OutDataTypeStr=boolean
  Unit Delay : UnitDelay  SampleTime=-1
  Unit Delay1 : UnitDelay  InitialCondition=1  SampleTime=-1
  Q : Outport
  !Q : Outport  Port=2
  wires:
  Logical Operator/1 -> Unit Delay1/1, !Q/1
  Logical Operator1/1 -> Unit Delay/1, Q/1
  Unit Delay/1 -> Logical Operator/1
  Unit Delay1/1 -> Logical Operator1/2
  Logical Operator2/1 -> Logical Operator1/1
  Logical Operator3/1 -> Logical Operator/2
  R/1 -> Logical Operator3/1
  S/1 -> Logical Operator2/1

== system Mode_plus_Longitudinal/LONGITUDINAL_CONTROLLER/Altitude Control/Variable Rate Limit/Variable Limit Saturation ==
  up_lim : Inport  RequirementInfo={} %GIDa_8fc29a2c_9a06_4d22_b2f8_ac29a6339ebb
  SigIn : Inport  RequirementInfo={} %GIDa_523f2031_cc7c_49a9_b970_4127022b0ac8  Port=2
  Lo_lim : Inport  RequirementInfo={} %GIDa_90811a43_da08_4eba_9b06_fee8f071624f  Port=3
  Enforce low lim : MinMax  RequirementInfo={} %GIDa_8232b52a_4d55_44bf_bb2a_0552ffc47f45  Function=max  Inputs=2
  Enforce up lim : MinMax  RequirementInfo={} %GIDa_7f73aa2d_fa36_44e6_8696_2eca4632477d  Inputs=2
  Out1 : Outport  RequirementInfo={} %GIDa_e741319d_3876_444b_80dd_e81dc2dc2ea4
  wires:
  Enforce up lim/1 -> Out1/1
  up_lim/1 -> Enforce up lim/2
  Enforce low lim/1 -> Enforce up lim/1
  SigIn/1 -> Enforce low lim/2
  Lo_lim/1 -> Enforce low lim/1

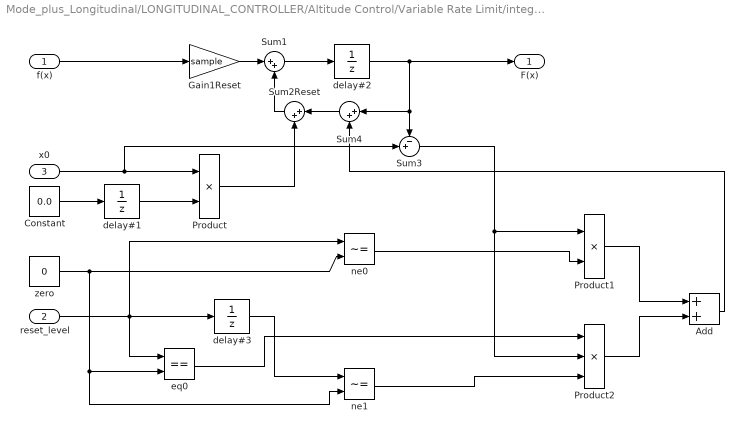
== system Mode_plus_Longitudinal/LONGITUDINAL_CONTROLLER/Altitude Control/Variable Rate Limit/integrator_reset ==
  f(x) : Inport  OutDataTypeStr=double  PortDimensions=1  SampleTime=sample
  reset_level : Inport  Port=2  OutDataTypeStr=boolean  PortDimensions=1  SampleTime=sample
  x0 : Inport  Port=3  OutDataTypeStr=double  PortDimensions=1  SampleTime=sample
  Add : Sum
  Constant : Constant  Value=0.0  SampleTime=sample
  Gain1Reset : Gain  RequirementInfo={} %GIDa_b9c0f26f_2220_4264_a2a6_639b1c650185  Gain=sample
  Product : Product  RndMeth=Zero
  Product1 : Product  OutDataTypeStr=double  RndMeth=Zero
  Product2 : Product  Inputs=3  OutDataTypeStr=double  RndMeth=Zero
  Sum1 : Sum  RequirementInfo={} %GIDa_0320a4df_befb_45fd_b671_d08bfe546209  Inputs=|++
  Sum2Reset : Sum  RequirementInfo={} %GIDa_83b52aad_626e_4978_a5cf_6b84b97897b3  Inputs=|++
  Sum3 : Sum  RequirementInfo={} %GIDa_babdad19_19c3_484f_b383_b2c6ad817b26  Inputs=-+|
  Sum4 : Sum  RequirementInfo={} %GIDa_1949a618_cee5_4978_84d2_096ea6f9b511  Inputs=|++
  delay#1 : UnitDelay  InitialCondition=1.0  SampleTime=-1
  delay#2 : UnitDelay  InitialCondition=0.0  SampleTime=-1
  delay#3 : UnitDelay  InitialCondition=0.0  SampleTime=-1
  eq0 : RelationalOperator  Operator===  OutDataTypeStr=boolean
  ne0 : RelationalOperator  Operator=~=  OutDataTypeStr=boolean
  ne1 : RelationalOperator  Operator=~=  OutDataTypeStr=boolean
  zero : Constant  Value=0  SampleTime=sample
  F(x) : Outport  RequirementInfo={} %GIDa_750a5e8d_483c_4826_9b6c_6a65252e8795
  wires:
  Sum1/1 -> delay#2/1
  Gain1Reset/1 -> Sum1/1
  delay#2/1 -> F(x)/1, Sum3/1, Sum4/1
  Sum2Reset/1 -> Sum1/2
  Product/1 -> Sum2Reset/2
  delay#1/1 -> Product/2
  Constant/1 -> delay#1/1
  f(x)/1 -> Gain1Reset/1
  x0/1 -> Product/1, Sum3/2
  reset_level/1 -> delay#3/1, ne0/1, eq0/1
  delay#3/1 -> ne1/1
  Sum3/1 -> Product1/1, Product2/2
  ne0/1 -> Product1/2
  eq0/1 -> Product2/1
  Product1/1 -> Add/1
  Product2/1 -> Add/2
  zero/1 -> ne0/2, eq0/2, ne1/2
  ne1/1 -> Product2/3
  Sum4/1 -> Sum2Reset/1
  Add/1 -> Sum4/2

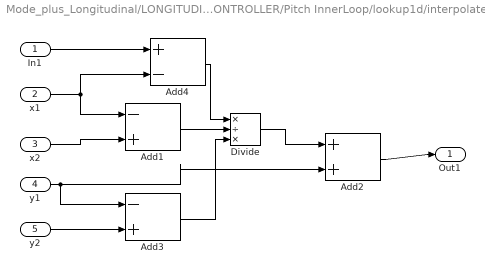
== system Mode_plus_Longitudinal/LONGITUDINAL_CONTROLLER/Pitch InnerLoop/lookup1d/interpolate1d#0 ==
  In1 : Inport
  x1 : Inport  Port=2
  x2 : Inport  Port=3
  y1 : Inport  Port=4
  y2 : Inport  Port=5
  Add1 : Sum  Inputs=-+
  Add2 : Sum
  Add3 : Sum  Inputs=-+
  Add4 : Sum  Inputs=+-
  Divide : Product  Inputs=*/*
  Out1 : Outport
  wires:
  Add2/1 -> Out1/1
  y1/1 -> Add2/2, Add3/1
  x2/1 -> Add1/2
  x1/1 -> Add1/1, Add4/2
  Add1/1 -> Divide/2
  y2/1 -> Add3/2
  Add3/1 -> Divide/3
  Divide/1 -> Add2/1
  Add4/1 -> Divide/1
  In1/1 -> Add4/1

== system Mode_plus_Longitudinal/LONGITUDINAL_CONTROLLER/Pitch InnerLoop/lookup1d/interpolate1d#1 ==
  In1 : Inport
  x1 : Inport  Port=2
  x2 : Inport  Port=3
  y1 : Inport  Port=4
  y2 : Inport  Port=5
  Add1 : Sum  Inputs=-+
  Add2 : Sum
  Add3 : Sum  Inputs=-+
  Add4 : Sum  Inputs=+-
  Divide : Product  Inputs=*/*
  Out1 : Outport
  wires:
  Add2/1 -> Out1/1
  y1/1 -> Add2/2, Add3/1
  x2/1 -> Add1/2
  x1/1 -> Add1/1, Add4/2
  Add1/1 -> Divide/2
  y2/1 -> Add3/2
  Add3/1 -> Divide/3
  Divide/1 -> Add2/1
  Add4/1 -> Divide/1
  In1/1 -> Add4/1

== system Mode_plus_Longitudinal/LONGITUDINAL_CONTROLLER/Pitch InnerLoop/lookup1d/interpolate1d#2 ==
  In1 : Inport
  x1 : Inport  Port=2
  x2 : Inport  Port=3
  y1 : Inport  Port=4
  y2 : Inport  Port=5
  Add1 : Sum  Inputs=-+
  Add2 : Sum
  Add3 : Sum  Inputs=-+
  Add4 : Sum  Inputs=+-
  Divide : Product  Inputs=*/*
  Out1 : Outport
  wires:
  Add2/1 -> Out1/1
  y1/1 -> Add2/2, Add3/1
  x2/1 -> Add1/2
  x1/1 -> Add1/1, Add4/2
  Add1/1 -> Divide/2
  y2/1 -> Add3/2
  Add3/1 -> Divide/3
  Divide/1 -> Add2/1
  Add4/1 -> Divide/1
  In1/1 -> Add4/1
